simulink model "example_controller_simulink"  (R2019b)
settings: Solver=VariableStepAuto  StartTime=0.0  StopTime=10.0  RelTol=1e-3
undefined symbols (not defined in the file): pose
libraries: ros2lib x3
settings Model: Creator=rc13011  LastModifiedBy=rc13011

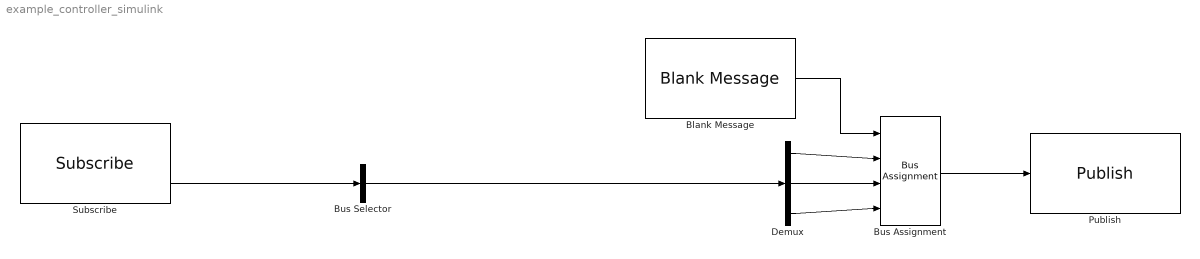
== system example_controller_simulink ==
  Blank Message : ros2lib/Blank Message  messageType=geometry_msgs/PoseStamped  SampleTime=inf
      settings: SourceProductName=ROS Toolbox  SourceProductBaseCode=RR
  Bus Assignment : BusAssignment  AssignedSignals=pose.position.x,pose.position.y,pose.position.z
  Bus Selector : BusSelector  OutputSignals=pose.position.x,pose.position.y,pose.position.z  OutputAsBus=on
  Demux : Demux  Outputs=3
  Publish : ros2lib/Publish  topicSource=Specify your own  topic=/mavros/setpoint_position/local  messageType=geometry_msgs/PoseStamped  QOSHistory=Keep last  QOSDepth=1  QOSReliability=Reliable  QOSDurability=Volatile
      settings: SourceProductName=ROS Toolbox  SourceProductBaseCode=RR
  Subscribe : ros2lib/Subscribe  topicSource=Specify your own  topic=/mavros/local_position/pose  messageType=geometry_msgs/PoseStamped  sampleTime=-1  QOSHistory=Keep last  QOSDepth=1  QOSReliability=Reliable  QOSDurability=Volatile
      settings: SourceProductName=ROS Toolbox  SourceProductBaseCode=RR
  wires:
  Subscribe/2 -> Bus Selector/1
  Bus Assignment/1 -> Publish/1
  Blank Message/1 -> Bus Assignment/1
  Demux/2 -> Bus Assignment/3
  Demux/1 -> Bus Assignment/2
  Demux/3 -> Bus Assignment/4
  Bus Selector/1 -> Demux/1
